simulink model "quad_to_mission_planner"  (R2024b)
settings: Solver=ode1  StartTime=0.0  StopTime=inf  FixedStep=0.01  RelTol=1e-3
undefined symbols (not defined in the file): Payload
libraries: uavmavlinklib x6, slpidlib x4, dspnetwork x3, simulink x2, uavutilslib x1
settings Model: Creator=ercu  LastModifiedBy=ercu
settings OptimizationCC: DefaultParameterBehavior=Inlined  EnhancedBackFolding=on  PassReuseOutputArgsAs=Individual arguments  ZeroExternalMemoryAtStartup=off  ZeroInternalMemoryAtStartup=off  OptimizeBlockOrder=speed  DifferentSizesBufferReuse=on  OptimizationCustomize=off  EfficientTunableParamExpr=on
settings DebuggingCC: ParameterTunabilityLossMsg=error
settings SFSimCC: MATLABDynamicMemAlloc=off
settings RTWCC: Description=Embedded Coder  SystemTargetFile=ert.tlc  GenCodeOnly=on  TemplateMakefile=ert_default_tmf  TargetLang=C++
settings CodeAppCC: ForceParamTrailComments=on  IgnoreCustomStorageClasses=off  OperatorAnnotations=on  SimulinkDataObjDesc=on  SFDataObjDesc=on  InsertBlockDesc=on
settings ERTTargetCC: TargetLangStandard=C++11 (ISO)  GenerateSampleERTMain=on  CodeInterfacePackaging=C++ class  RootIOFormat=Structure reference  ERTCustomFileTemplate=example_file_process.tlc

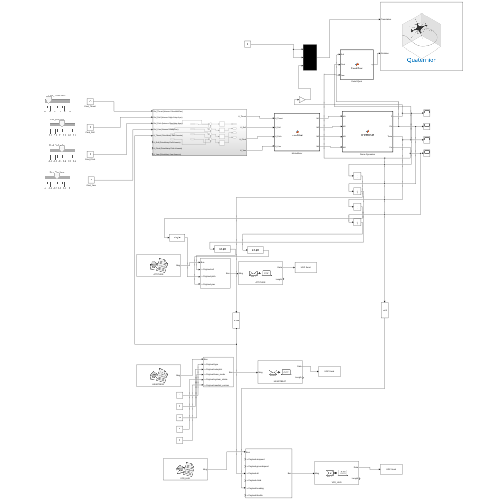
[thumbnail: Simulink's stored preview of the top-level diagram]
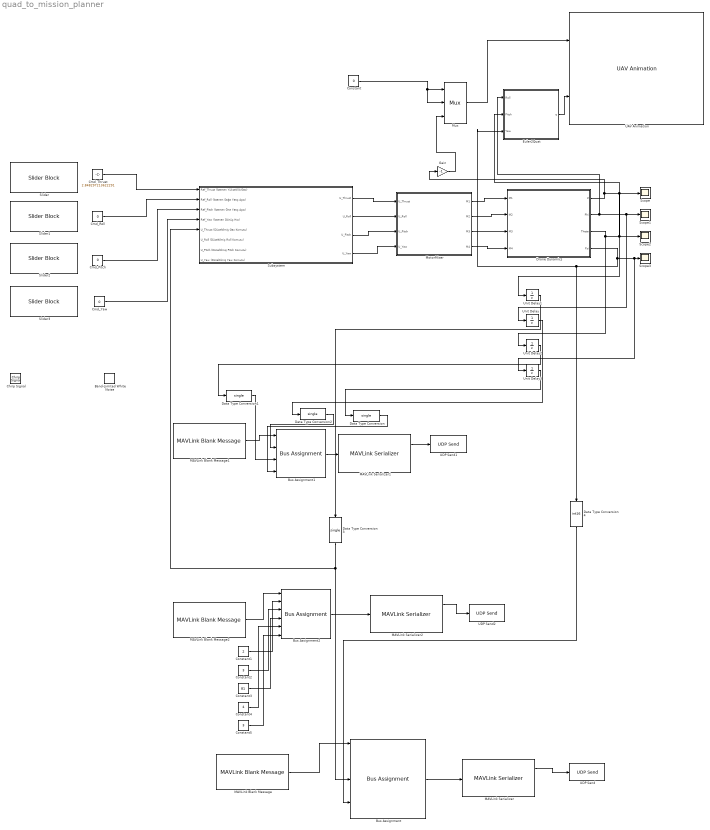
== system quad_to_mission_planner ==
  Bus Assignment : BusAssignment  AssignedSignals=Payload.airspeed,Payload.groundspeed,Payload.alt,Payload.climb,Payload.heading,Payload.throttle
  Bus Assignment1 : BusAssignment  AssignedSignals=Payload.roll,Payload.pitch,Payload.yaw
  Bus Assignment2 : BusAssignment  AssignedSignals=Payload.type,Payload.autopilot,Payload.base_mode,Payload.system_status,Payload.mavlink_version
  Cmd_Pitch : Constant  Value=0
  Cmd_Roll : Constant  Value=0
  Cmd_Thrust : Constant  Value=2.848297213622291
  Cmd_Yaw : Constant  Value=0
  Constant : Constant  Value=0
  Constant1 : Constant  Value=2  OutDataTypeStr=uint8
  Constant2 : Constant  Value=3  OutDataTypeStr=uint8
  Constant3 : Constant  Value=81  OutDataTypeStr=uint8
  Constant4 : Constant  Value=4  OutDataTypeStr=uint8
  Constant5 : Constant  Value=3  OutDataTypeStr=uint8
  Data Type Conversion{,1..3} (4 alike) : DataTypeConversion  OutDataTypeStr=single  SaturateOnIntegerOverflow=off  RndMeth=Floor
  Data Type Conversion4 : DataTypeConversion  OutDataTypeStr=int16  SaturateOnIntegerOverflow=off  RndMeth=Floor
  Drone Dynamics : MATLAB Function  TreatAsAtomicUnit=on
  Euler2Quat : MATLAB Function  TreatAsAtomicUnit=on
  Gain : Gain  Gain=-1
  MAVLink Blank Message : uavmavlinklib/MAVLink Blank Message  dialectSource=Select from standard MAVLink dialects  dialect=common.xml  dialectCustom=common.xml  version=2  messageType=VFR_HUD  SystemID=1  ComponentID=1  SampleTime=inf
  MAVLink Blank Message1 : uavmavlinklib/MAVLink Blank Message  dialectSource=Select from standard MAVLink dialects  dialect=common.xml  dialectCustom=common.xml  version=2  messageType=ATTITUDE  SystemID=1  ComponentID=1  SampleTime=inf
  MAVLink Blank Message2 : uavmavlinklib/MAVLink Blank Message  dialectSource=Select from standard MAVLink dialects  dialect=common.xml  dialectCustom=common.xml  version=2  messageType=HEARTBEAT  SystemID=1  ComponentID=1  SampleTime=inf
  MAVLink Serializer : uavmavlinklib/MAVLink Serializer  dialectSource=Select from standard MAVLink dialects  dialect=common.xml  dialectCustom=common.xml  version=2  messageType=VFR_HUD
  MAVLink Serializer1 : uavmavlinklib/MAVLink Serializer  dialectSource=Select from standard MAVLink dialects  dialect=common.xml  dialectCustom=common.xml  version=2  messageType=ATTITUDE
  MAVLink Serializer2 : uavmavlinklib/MAVLink Serializer  dialectSource=Select from standard MAVLink dialects  dialect=common.xml  dialectCustom=common.xml  version=2  messageType=HEARTBEAT
  MotorMixer : MATLAB Function  TreatAsAtomicUnit=on
  Mux : Mux  Inputs=3
  Scope{,1..3} (4 alike) : Scope
  Slider : SliderBlock  ScaleMax=20
  Slider1 : SliderBlock  ScaleMin=-0.5  ScaleMax=0.5
  Slider2 : SliderBlock  ScaleMin=-0.5  ScaleMax=0.5
  Slider3 : SliderBlock  ScaleMin=-1  ScaleMax=1
  Subsystem : Subsystem
  UAV Animation : uavutilslib/UAV Animation  NumUAV=1  DynamicUAVConfig=off  UAVType=Multirotor  UAVSize=1  UAVColor=[1 0 0]  UAVTrajectoryAlpha=1  InertialZDirection=Down  RotationFormat=Quaternion  DrawMarkers=off  SampleTime=-1
  UDP Send : dspnetwork/UDP Send  remoteURL='127.0.0.1'  remotePort=14550  localURL='0.0.0.0'  localPortSource=Automatically determine  localPort=-1  sendBufferSize=8192  sampletime=-1  blockPlatform=[]  separateLengthPort=0
      settings: LibrarySourceBlock=dspsnks4/UDP Send
  UDP Send1 : dspnetwork/UDP Send  remoteURL='127.0.0.1'  remotePort=14550  localURL='0.0.0.0'  localPortSource=Automatically determine  localPort=-1  sendBufferSize=8192  sampletime=-1  blockPlatform=[]  separateLengthPort=0
      settings: LibrarySourceBlock=dspsnks4/UDP Send
  UDP Send2 : dspnetwork/UDP Send  remoteURL='127.0.0.1'  remotePort=14550  localURL='0.0.0.0'  localPortSource=Automatically determine  localPort=-1  sendBufferSize=8192  sampletime=-1  blockPlatform=[]  separateLengthPort=0
      settings: LibrarySourceBlock=dspsnks4/UDP Send
  Unit Delay{,1..3} (4 alike) : UnitDelay  SampleTime=-1  HasFrameUpgradeWarning=on
  Band-Limited White Noise : simulink/Sources/Band-Limited White Noise  IOType=siggen  Cov=[0.1]  Ts=0.1  seed=[23341]
      settings: LibrarySourceBlock=|
      | simgens/Band-Limited
      | White Noise
  Chirp Signal : simulink/Sources/Chirp Signal  IOType=siggen  f1=0.1  T=100  f2=1
      settings: LibrarySourceBlock=simgens/Chirp Signal
  wires:
  Bus Assignment1/1 -> MAVLink Serializer1/1
  MAVLink Blank Message1/1 -> Bus Assignment1/1
  MAVLink Serializer1/1 -> UDP Send1/1
  Drone Dynamics/3(Theta) -> Unit Delay2/1, Euler2Quat/2(Pitch), Scope2/1
  Drone Dynamics/1(Z) -> Gain/1, Unit Delay1/1, Scope/1
  Unit Delay3/1 -> Data Type Conversion/1
  Unit Delay2/1 -> Data Type Conversion1/1
  MotorMixer/1(M1) -> Drone Dynamics/1(M1)
  Unit Delay/1 -> Data Type Conversion2/1
  Constant/1 -> Mux/2, Mux/1
  Subsystem/1(U_Thrust) -> MotorMixer/1(U_Thrust)
  Euler2Quat/1(q) -> UAV Animation/2
  MotorMixer/3(M3) -> Drone Dynamics/3(M3)
  Drone Dynamics/2(Phi) -> Euler2Quat/1(Roll), Unit Delay/1, Scope1/1
  Subsystem/2(U_Roll) -> MotorMixer/2(U_Roll)
  Mux/1 -> UAV Animation/1
  MotorMixer/4(M4) -> Drone Dynamics/4(M4)
  Cmd_Roll/1 -> Subsystem/2(Ref_Roll (İstenen Sağa Yatış Açısı))
  Cmd_Yaw/1 -> Subsystem/4(Ref_Yaw (İstenen Dönüş Hızı))
  Subsystem/4(U_Yaw) -> MotorMixer/4(U_Yaw)
  Cmd_Pitch/1 -> Subsystem/3(Ref_Pitch (İstenen Öne Yatış Açısı))
  MotorMixer/2(M2) -> Drone Dynamics/2(M2)
  Unit Delay1/1 -> Data Type Conversion3/1
  Cmd_Thrust/1 -> Subsystem/1(Ref_Thrust (İstenen Yükseklik/Gaz))
  Gain/1 -> Mux/3
  Subsystem/3(U_Pitch) -> MotorMixer/3(U_Pitch)
  MAVLink Blank Message2/1 -> Bus Assignment2/1
  Constant1/1 -> Bus Assignment2/2
  Constant2/1 -> Bus Assignment2/3
  Constant3/1 -> Bus Assignment2/4
  Constant4/1 -> Bus Assignment2/5
  Constant5/1 -> Bus Assignment2/6
  Bus Assignment2/1 -> MAVLink Serializer2/1
  MAVLink Serializer2/1 -> UDP Send2/1
  MAVLink Blank Message/1 -> Bus Assignment/1
  Drone Dynamics/4(Psi) -> Euler2Quat/3(Yaw), Data Type Conversion4/1, Unit Delay3/1, Scope3/1
  Bus Assignment/1 -> MAVLink Serializer/1
  MAVLink Serializer/1 -> UDP Send/1
  Data Type Conversion4/1 -> Bus Assignment/6
  Data Type Conversion/1 -> Bus Assignment1/4
  Data Type Conversion1/1 -> Bus Assignment1/3
  Data Type Conversion2/1 -> Bus Assignment1/2
  Data Type Conversion3/1 -> Subsystem/5(U_Thrust (Düzeltilmiş Gaz Komutu)), Bus Assignment/4

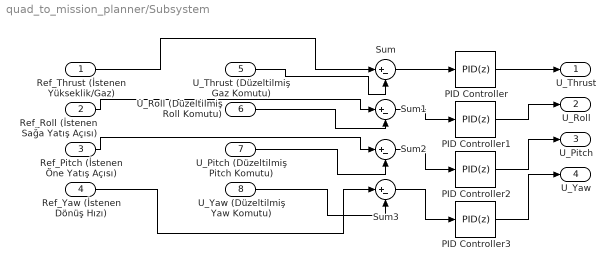
== system quad_to_mission_planner/Subsystem ==
  Ref_Thrust (İstenen Yükseklik/Gaz) : Inport
  Ref_Roll (İstenen Sağa Yatış Açısı) : Inport  Port=2
  Ref_Pitch (İstenen Öne Yatış Açısı) : Inport  Port=3
  Ref_Yaw (İstenen Dönüş Hızı) : Inport  Port=4
  U_Thrust (Düzeltilmiş Gaz Komutu) : Inport  Port=5
  U_Roll (Düzeltilmiş Roll Komutu) : Inport  Port=6
  U_Pitch (Düzeltilmiş Pitch Komutu) : Inport  Port=7
  U_Yaw (Düzeltilmiş Yaw Komutu) : Inport  Port=8
  PID Controller : slpidlib/PID Controller  Controller=PID  Form=Parallel  TimeDomain=Discrete-time  UseExternalTs=off  SampleTime=0.01  IntegratorMethod=Forward Euler  FilterMethod=Forward Euler  ControllerParametersSource=internal  P=3  I=1.5  UseKiTs=off  D=2.5  UseExternalDerivativeSource=off  N=100  UseFilter=on  TunerSelectOption=Transfer Function Based (PID Tuner App)  InitialConditionSource=internal  InitialConditionForIntegrator=0  InitialConditionForFilter=0  DifferentiatorICPrevScaledInput=0  ExternalReset=none  TrackingMode=off  Kt=1  LimitOutput=off  SatLimitsSource=internal  UpperSaturationLimit=inf  LowerSaturationLimit=-inf  LinearizeAsGain=on  AntiWindupMode=none  Kb=1  LimitIntegrator=off  UpperIntegratorSaturationLimit=inf  LowerIntegratorSaturationLimit=-inf  POutMin=[]  POutMax=[]  IOutMin=[]  IOutMax=[]  DOutMin=[]  DOutMax=[]  NOutMin=[]  NOutMax=[]  SumOutMin=[]  SumOutMax=[]  SaturationOutMin=[]  SaturationOutMax=[]  PParamMin=[]  PParamMax=[]  IParamMin=[]  IParamMax=[]  DParamMin=[]  DParamMax=[]  NParamMin=[]  NParamMax=[]  KbParamMin=[]  KbParamMax=[]  KtParamMin=[]  KtParamMax=[]  KbOutMin=[]  KbOutMax=[]  KtOutMin=[]  KtOutMax=[]  IntegratorOutMin=[]  IntegratorOutMax=[]  FilterOutMin=[]  FilterOutMax=[]  SumI1OutMin=[]  SumI1OutMax=[]  SumI2OutMin=[]  SumI2OutMax=[]  SumI3OutMin=[]  SumI3OutMax=[]  SumI4OutMin=[]  SumI4OutMax=[]  SumDOutMin=[]  SumDOutMax=[]  DifferentiatorOutMin=[]  DifferentiatorOutMax=[]  FilterDiffOutCoefMin=[]  FilterDiffOutCoefMax=[]  ReciprocalOutMin=[]  ReciprocalOutMax=[]  SumDenOutMin=[]  SumDenOutMax=[]  SumNumOutMin=[]  SumNumOutMax=[]  DivideOutMin=[]  DivideOutMax=[]  UdiffTsProdOutMin=[]  UdiffTsProdOutMax=[]  NTsProdOutMin=[]  NTsProdOutMax=[]  UintegralTsProdOutMin=[]  UintegralTsProdOutMax=[]  UngainTsProdOutMin=[]  UngainTsProdOutMax=[]  ClampingZeroOutDataTypeStr=Inherit: Inherit via back propagation  ClampingZeroOutMin=[]  ClampingZeroOutMax=[]  FilterDenConstantOutDataTypeStr=Inherit: Inherit via back propagation  FilterDenConstantOutMin=[]  FilterDenConstantOutMax=[]  PCopyOutDataTypeStr=Inherit: Inherit via back propagation  PCopyOutMin=[]  PCopyOutMax=[]  NCopyOutDataTypeStr=Inherit: Inherit via back propagation  NCopyOutMin=[]  NCopyOutMax=[]  IntegratorContinuousStateAttributes=''  IntegratorStateMustResolveToSignalObject=off  IntegratorRTWStateStorageClass=Auto  FilterContinuousStateAttributes=''  FilterStateMustResolveToSignalObject=off  FilterRTWStateStorageClass=Auto  ParallelPVariant=InternalParameters  IdealPVariant=Disabled  IVariant=InternalParameters  DVariant=InternalParameters  IntegratorVariant=Discrete  SatVariant=Disabled  AWVariant=Passthrough  PCopyVariant=Disabled  TRVariant=Disabled  FdbkBlocksVariant=Forward  IdealPFdbkVariant=Disabled  SatFdbkVariant=Disabled  DerivativeFilterVariant=ForwardEulerFilter  NVariant=InternalParameters  NCopyVariant=Disabled  FilterICVariant=InternalICsFilter  IntegratorICVariant=InternalICs  ExternalResetVariant=Disabled  TRSumVariant=Passthrough  SumFdbkVariant=Disabled  SumVariant=Sum_PID  TsampFilterVariant=InternalTs  TsampNgainVariant=Passthrough  TsampIntegralVariant=Disabled_SignalSpec  ExternalSaturationOutDataTypeStr=Inherit: Same as second input  DerivativeSourceVariant=ErrorSignal  PreIntVariant=InternalPreInt
  PID Controller1 : slpidlib/PID Controller  Controller=PID  Form=Parallel  TimeDomain=Discrete-time  UseExternalTs=off  SampleTime=0.01  IntegratorMethod=Forward Euler  FilterMethod=Forward Euler  ControllerParametersSource=internal  P=2  I=0  UseKiTs=off  D=0.5  UseExternalDerivativeSource=off  N=100  UseFilter=on  TunerSelectOption=Transfer Function Based (PID Tuner App)  InitialConditionSource=internal  InitialConditionForIntegrator=0  InitialConditionForFilter=0  DifferentiatorICPrevScaledInput=0  ExternalReset=none  TrackingMode=off  Kt=1  LimitOutput=off  SatLimitsSource=internal  UpperSaturationLimit=inf  LowerSaturationLimit=-inf  LinearizeAsGain=on  AntiWindupMode=none  Kb=1  LimitIntegrator=off  UpperIntegratorSaturationLimit=inf  LowerIntegratorSaturationLimit=-inf  POutMin=[]  POutMax=[]  IOutMin=[]  IOutMax=[]  DOutMin=[]  DOutMax=[]  NOutMin=[]  NOutMax=[]  SumOutMin=[]  SumOutMax=[]  SaturationOutMin=[]  SaturationOutMax=[]  PParamMin=[]  PParamMax=[]  IParamMin=[]  IParamMax=[]  DParamMin=[]  DParamMax=[]  NParamMin=[]  NParamMax=[]  KbParamMin=[]  KbParamMax=[]  KtParamMin=[]  KtParamMax=[]  KbOutMin=[]  KbOutMax=[]  KtOutMin=[]  KtOutMax=[]  IntegratorOutMin=[]  IntegratorOutMax=[]  FilterOutMin=[]  FilterOutMax=[]  SumI1OutMin=[]  SumI1OutMax=[]  SumI2OutMin=[]  SumI2OutMax=[]  SumI3OutMin=[]  SumI3OutMax=[]  SumI4OutMin=[]  SumI4OutMax=[]  SumDOutMin=[]  SumDOutMax=[]  DifferentiatorOutMin=[]  DifferentiatorOutMax=[]  FilterDiffOutCoefMin=[]  FilterDiffOutCoefMax=[]  ReciprocalOutMin=[]  ReciprocalOutMax=[]  SumDenOutMin=[]  SumDenOutMax=[]  SumNumOutMin=[]  SumNumOutMax=[]  DivideOutMin=[]  DivideOutMax=[]  UdiffTsProdOutMin=[]  UdiffTsProdOutMax=[]  NTsProdOutMin=[]  NTsProdOutMax=[]  UintegralTsProdOutMin=[]  UintegralTsProdOutMax=[]  UngainTsProdOutMin=[]  UngainTsProdOutMax=[]  ClampingZeroOutDataTypeStr=Inherit: Inherit via back propagation  ClampingZeroOutMin=[]  ClampingZeroOutMax=[]  FilterDenConstantOutDataTypeStr=Inherit: Inherit via back propagation  FilterDenConstantOutMin=[]  FilterDenConstantOutMax=[]  PCopyOutDataTypeStr=Inherit: Inherit via back propagation  PCopyOutMin=[]  PCopyOutMax=[]  NCopyOutDataTypeStr=Inherit: Inherit via back propagation  NCopyOutMin=[]  NCopyOutMax=[]  IntegratorContinuousStateAttributes=''  IntegratorStateMustResolveToSignalObject=off  IntegratorRTWStateStorageClass=Auto  FilterContinuousStateAttributes=''  FilterStateMustResolveToSignalObject=off  FilterRTWStateStorageClass=Auto  ParallelPVariant=InternalParameters  IdealPVariant=Disabled  IVariant=InternalParameters  DVariant=InternalParameters  IntegratorVariant=Discrete  SatVariant=Disabled  AWVariant=Passthrough  PCopyVariant=Disabled  TRVariant=Disabled  FdbkBlocksVariant=Forward  IdealPFdbkVariant=Disabled  SatFdbkVariant=Disabled  DerivativeFilterVariant=ForwardEulerFilter  NVariant=InternalParameters  NCopyVariant=Disabled  FilterICVariant=InternalICsFilter  IntegratorICVariant=InternalICs  ExternalResetVariant=Disabled  TRSumVariant=Passthrough  SumFdbkVariant=Disabled  SumVariant=Sum_PID  TsampFilterVariant=InternalTs  TsampNgainVariant=Passthrough  TsampIntegralVariant=Disabled_SignalSpec  ExternalSaturationOutDataTypeStr=Inherit: Same as second input  DerivativeSourceVariant=ErrorSignal  PreIntVariant=InternalPreInt
  PID Controller2 : slpidlib/PID Controller  Controller=PID  Form=Parallel  TimeDomain=Discrete-time  UseExternalTs=off  SampleTime=0.01  IntegratorMethod=Forward Euler  FilterMethod=Forward Euler  ControllerParametersSource=internal  P=2  I=0  UseKiTs=off  D=0.5  UseExternalDerivativeSource=off  N=100  UseFilter=on  TunerSelectOption=Transfer Function Based (PID Tuner App)  InitialConditionSource=internal  InitialConditionForIntegrator=0  InitialConditionForFilter=0  DifferentiatorICPrevScaledInput=0  ExternalReset=none  TrackingMode=off  Kt=1  LimitOutput=off  SatLimitsSource=internal  UpperSaturationLimit=inf  LowerSaturationLimit=-inf  LinearizeAsGain=on  AntiWindupMode=none  Kb=1  LimitIntegrator=off  UpperIntegratorSaturationLimit=inf  LowerIntegratorSaturationLimit=-inf  POutMin=[]  POutMax=[]  IOutMin=[]  IOutMax=[]  DOutMin=[]  DOutMax=[]  NOutMin=[]  NOutMax=[]  SumOutMin=[]  SumOutMax=[]  SaturationOutMin=[]  SaturationOutMax=[]  PParamMin=[]  PParamMax=[]  IParamMin=[]  IParamMax=[]  DParamMin=[]  DParamMax=[]  NParamMin=[]  NParamMax=[]  KbParamMin=[]  KbParamMax=[]  KtParamMin=[]  KtParamMax=[]  KbOutMin=[]  KbOutMax=[]  KtOutMin=[]  KtOutMax=[]  IntegratorOutMin=[]  IntegratorOutMax=[]  FilterOutMin=[]  FilterOutMax=[]  SumI1OutMin=[]  SumI1OutMax=[]  SumI2OutMin=[]  SumI2OutMax=[]  SumI3OutMin=[]  SumI3OutMax=[]  SumI4OutMin=[]  SumI4OutMax=[]  SumDOutMin=[]  SumDOutMax=[]  DifferentiatorOutMin=[]  DifferentiatorOutMax=[]  FilterDiffOutCoefMin=[]  FilterDiffOutCoefMax=[]  ReciprocalOutMin=[]  ReciprocalOutMax=[]  SumDenOutMin=[]  SumDenOutMax=[]  SumNumOutMin=[]  SumNumOutMax=[]  DivideOutMin=[]  DivideOutMax=[]  UdiffTsProdOutMin=[]  UdiffTsProdOutMax=[]  NTsProdOutMin=[]  NTsProdOutMax=[]  UintegralTsProdOutMin=[]  UintegralTsProdOutMax=[]  UngainTsProdOutMin=[]  UngainTsProdOutMax=[]  ClampingZeroOutDataTypeStr=Inherit: Inherit via back propagation  ClampingZeroOutMin=[]  ClampingZeroOutMax=[]  FilterDenConstantOutDataTypeStr=Inherit: Inherit via back propagation  FilterDenConstantOutMin=[]  FilterDenConstantOutMax=[]  PCopyOutDataTypeStr=Inherit: Inherit via back propagation  PCopyOutMin=[]  PCopyOutMax=[]  NCopyOutDataTypeStr=Inherit: Inherit via back propagation  NCopyOutMin=[]  NCopyOutMax=[]  IntegratorContinuousStateAttributes=''  IntegratorStateMustResolveToSignalObject=off  IntegratorRTWStateStorageClass=Auto  FilterContinuousStateAttributes=''  FilterStateMustResolveToSignalObject=off  FilterRTWStateStorageClass=Auto  ParallelPVariant=InternalParameters  IdealPVariant=Disabled  IVariant=InternalParameters  DVariant=InternalParameters  IntegratorVariant=Discrete  SatVariant=Disabled  AWVariant=Passthrough  PCopyVariant=Disabled  TRVariant=Disabled  FdbkBlocksVariant=Forward  IdealPFdbkVariant=Disabled  SatFdbkVariant=Disabled  DerivativeFilterVariant=ForwardEulerFilter  NVariant=InternalParameters  NCopyVariant=Disabled  FilterICVariant=InternalICsFilter  IntegratorICVariant=InternalICs  ExternalResetVariant=Disabled  TRSumVariant=Passthrough  SumFdbkVariant=Disabled  SumVariant=Sum_PID  TsampFilterVariant=InternalTs  TsampNgainVariant=Passthrough  TsampIntegralVariant=Disabled_SignalSpec  ExternalSaturationOutDataTypeStr=Inherit: Same as second input  DerivativeSourceVariant=ErrorSignal  PreIntVariant=InternalPreInt
  PID Controller3 : slpidlib/PID Controller  Controller=PID  Form=Parallel  TimeDomain=Discrete-time  UseExternalTs=off  SampleTime=0.01  IntegratorMethod=Forward Euler  FilterMethod=Forward Euler  ControllerParametersSource=internal  P=4  I=0.5  UseKiTs=off  D=0  UseExternalDerivativeSource=off  N=100  UseFilter=on  TunerSelectOption=Transfer Function Based (PID Tuner App)  InitialConditionSource=internal  InitialConditionForIntegrator=0  InitialConditionForFilter=0  DifferentiatorICPrevScaledInput=0  ExternalReset=none  TrackingMode=off  Kt=1  LimitOutput=off  SatLimitsSource=internal  UpperSaturationLimit=inf  LowerSaturationLimit=-inf  LinearizeAsGain=on  AntiWindupMode=none  Kb=1  LimitIntegrator=off  UpperIntegratorSaturationLimit=inf  LowerIntegratorSaturationLimit=-inf  POutMin=[]  POutMax=[]  IOutMin=[]  IOutMax=[]  DOutMin=[]  DOutMax=[]  NOutMin=[]  NOutMax=[]  SumOutMin=[]  SumOutMax=[]  SaturationOutMin=[]  SaturationOutMax=[]  PParamMin=[]  PParamMax=[]  IParamMin=[]  IParamMax=[]  DParamMin=[]  DParamMax=[]  NParamMin=[]  NParamMax=[]  KbParamMin=[]  KbParamMax=[]  KtParamMin=[]  KtParamMax=[]  KbOutMin=[]  KbOutMax=[]  KtOutMin=[]  KtOutMax=[]  IntegratorOutMin=[]  IntegratorOutMax=[]  FilterOutMin=[]  FilterOutMax=[]  SumI1OutMin=[]  SumI1OutMax=[]  SumI2OutMin=[]  SumI2OutMax=[]  SumI3OutMin=[]  SumI3OutMax=[]  SumI4OutMin=[]  SumI4OutMax=[]  SumDOutMin=[]  SumDOutMax=[]  DifferentiatorOutMin=[]  DifferentiatorOutMax=[]  FilterDiffOutCoefMin=[]  FilterDiffOutCoefMax=[]  ReciprocalOutMin=[]  ReciprocalOutMax=[]  SumDenOutMin=[]  SumDenOutMax=[]  SumNumOutMin=[]  SumNumOutMax=[]  DivideOutMin=[]  DivideOutMax=[]  UdiffTsProdOutMin=[]  UdiffTsProdOutMax=[]  NTsProdOutMin=[]  NTsProdOutMax=[]  UintegralTsProdOutMin=[]  UintegralTsProdOutMax=[]  UngainTsProdOutMin=[]  UngainTsProdOutMax=[]  ClampingZeroOutDataTypeStr=Inherit: Inherit via back propagation  ClampingZeroOutMin=[]  ClampingZeroOutMax=[]  FilterDenConstantOutDataTypeStr=Inherit: Inherit via back propagation  FilterDenConstantOutMin=[]  FilterDenConstantOutMax=[]  PCopyOutDataTypeStr=Inherit: Inherit via back propagation  PCopyOutMin=[]  PCopyOutMax=[]  NCopyOutDataTypeStr=Inherit: Inherit via back propagation  NCopyOutMin=[]  NCopyOutMax=[]  IntegratorContinuousStateAttributes=''  IntegratorStateMustResolveToSignalObject=off  IntegratorRTWStateStorageClass=Auto  FilterContinuousStateAttributes=''  FilterStateMustResolveToSignalObject=off  FilterRTWStateStorageClass=Auto  ParallelPVariant=InternalParameters  IdealPVariant=Disabled  IVariant=InternalParameters  DVariant=InternalParameters  IntegratorVariant=Discrete  SatVariant=Disabled  AWVariant=Passthrough  PCopyVariant=Disabled  TRVariant=Disabled  FdbkBlocksVariant=Forward  IdealPFdbkVariant=Disabled  SatFdbkVariant=Disabled  DerivativeFilterVariant=ForwardEulerFilter  NVariant=InternalParameters  NCopyVariant=Disabled  FilterICVariant=InternalICsFilter  IntegratorICVariant=InternalICs  ExternalResetVariant=Disabled  TRSumVariant=Passthrough  SumFdbkVariant=Disabled  SumVariant=Sum_PID  TsampFilterVariant=InternalTs  TsampNgainVariant=Passthrough  TsampIntegralVariant=Disabled_SignalSpec  ExternalSaturationOutDataTypeStr=Inherit: Same as second input  DerivativeSourceVariant=ErrorSignal  PreIntVariant=InternalPreInt
  Sum{,1..3} (4 alike) : Sum  Inputs=|+-
  U_Thrust : Outport
  U_Roll : Outport  Port=2
  U_Pitch : Outport  Port=3
  U_Yaw : Outport  Port=4
  wires:
  Ref_Thrust (İstenen Yükseklik/Gaz)/1 -> Sum/1
  Ref_Roll (İstenen Sağa Yatış Açısı)/1 -> Sum1/1
  Ref_Pitch (İstenen Öne Yatış Açısı)/1 -> Sum2/1
  Ref_Yaw (İstenen Dönüş Hızı)/1 -> Sum3/1
  U_Pitch (Düzeltilmiş Pitch Komutu)/1 -> Sum2/2
  U_Roll (Düzeltilmiş Roll Komutu)/1 -> Sum1/2
  U_Thrust (Düzeltilmiş Gaz Komutu)/1 -> Sum/2
  Sum/1 -> PID Controller/1
  Sum1/1 -> PID Controller1/1
  Sum2/1 -> PID Controller2/1
  Sum3/1 -> PID Controller3/1
  PID Controller/1 -> U_Thrust/1
  PID Controller1/1 -> U_Roll/1
  PID Controller2/1 -> U_Pitch/1
  PID Controller3/1 -> U_Yaw/1
  U_Yaw (Düzeltilmiş Yaw Komutu)/1 -> Sum3/2

== matlab function quad_to_mission_planner/Drone Dynamics ==
  data: M1 input; Z output; M2 input; M3 input; M4 input; Phi output; Theta output; Psi output
function [Z, Phi, Theta, Psi] = DronePhysics(M1, M2, M3, M4)
    % Drone Fizigi - ACI KONTROL MODU (Angle Control)
    % Z: Yukseklik, Phi: Roll, Theta: Pitch, Psi: Yaw
    
    persistent p_Z p_Phi p_Theta p_Psi v_Z v_Phi v_Theta v_Psi
    
    if isempty(p_Z)
        p_Z=0; p_Phi=0; p_Theta=0; p_Psi=0;
        v_Z=0; v_Phi=0; v_Theta=0; v_Psi=0;
    end
    
    dt = 0.01; 
    m = 1.2;   
    g = 9.81;
    Ixx = 0.01; Iyy = 0.01; Izz = 0.02; 
    
    % Kuvvetler
    F_total = M1 + M2 + M3 + M4;
    Tau_Roll = (M2 + M3) - (M1 + M4); 
    Tau_Pitch = (M1 + M3) - (M2 + M4); 
    Tau_Yaw = (M1 + M2) - (M3 + M4); 
    
    % --- SURTUNME (DAMPING) ---
    % Dronun donusunu yavaslatmak icin sart
    b_rot = 0.5; 
    
    % 1. Z Ekseni
    acc_Z = (F_total / m) - g;
    v_Z = v_Z + acc_Z * dt;
    p_Z = p_Z + v_Z * dt;
    if p_Z < 0; p_Z = 0; v_Z = 0; end 
    
    % 2. Acisal Hareket (Surtunmeli)
    alpha_Roll = (Tau_Roll - (v_Phi * b_rot)) / Ixx;
    alpha_Pitch = (Tau_Pitch - (v_Theta * b_rot)) / Iyy;
    alpha_Yaw = (Tau_Yaw - (v_Psi * b_rot)) / Izz;
    
    % Integrasyon
    v_Phi = v_Phi + alpha_Roll * dt;
    p_Phi = p_Phi + v_Phi * dt;
    
    v_Theta = v_Theta + alpha_Pitch * dt;
    p_Theta = p_Theta + v_Theta * dt;
    
    v_Psi = v_Psi + alpha_Yaw * dt;
    p_Psi = p_Psi + v_Psi * dt;
    
    % Cikislar (Sadece Acilar)
    Z = p_Z;
    Phi = p_Phi;
    Theta = p_Theta;
    Psi = p_Psi; 
end

== matlab function quad_to_mission_planner/MotorMixer ==
  data: U_Thrust input; M1 output; U_Roll input; U_Pitch input; U_Yaw input; M2 output; M3 output; M4 output
function [M1, M2, M3, M4] = MotorMixer(U_Thrust, U_Roll, U_Pitch, U_Yaw)
    % Quadcopter X Config Motor Mixing Algorithm
    % M1: Sag On (CCW), M2: Sol Arka (CCW) -> Tersi yonler
    % M3: Sol On (CW),  M4: Sag Arka (CW)
    
    % Temel Mantik:
    % Roll sag istiyorsa -> Sol motorlari artir, Sag motorlari azalt.
    % Pitch on istiyorsa -> Arka motorlari artir, On motorlari azalt.
    
    % Mixing Matrix
    M1 = U_Thrust - U_Roll + U_Pitch + U_Yaw; % Sag On
    M2 = U_Thrust + U_Roll - U_Pitch + U_Yaw; % Sol Arka
    M3 = U_Thrust + U_Roll + U_Pitch - U_Yaw; % Sol On
    M4 = U_Thrust - U_Roll - U_Pitch - U_Yaw; % Sag Arka
    
    % Motor Limitleri (Saturation)
    % Motorlar eksi donemez, max 30N uretebilir
    M1 = min(max(M1, 0), 30);
    M2 = min(max(M2, 0), 30);
    M3 = min(max(M3, 0), 30);
    M4 = min(max(M4, 0), 30);
end

== matlab function quad_to_mission_planner/Euler2Quat ==
  data: Roll input; q output; Pitch input; Yaw input
function q = Euler2Quat(Roll, Pitch, Yaw)
    % Simulink Code Gen uyumlu Manuel Donusum
    % Euler ZYX Siralamasi (Yaw -> Pitch -> Roll)
    
    % Yari acilarin cos ve sin degerleri
    c1 = cos(Yaw / 2);
    s1 = sin(Yaw / 2);
    c2 = cos(Pitch / 2);
    s2 = sin(Pitch / 2);
    c3 = cos(Roll / 2);
    s3 = sin(Roll / 2);

    % Quaternion bilesenleri (w, x, y, z)
    w = c1 * c2 * c3 + s1 * s2 * s3;
    x = c1 * c2 * s3 - s1 * s2 * c3;
    y = c1 * s2 * c3 + s1 * c2 * s3;
    z = s1 * c2 * c3 - c1 * s2 * s3;

    % Cikis vektoru (1x4)
    q = [w, x, y, z];
end
